simulink model "ADC_DAC_SimulinkModel_2016a"  (R2016a)
settings: Solver=VariableStepDiscrete  StartTime=0.0  StopTime=(2*N-1)/fs  FixedStep=1/fs  RelTol=1e-3
values from neighbouring files (symbols this model uses):
  AmpSig = 0.49    [DAC_Model_Analysis.m]
  fin = k*fs/N    [DAC_Model_Analysis.m]
  fs = 200e6    (= 200000000)    [DAC_Model_Analysis.m]
  gain = 1    [DAC_Model_Analysis.m]
  jitter = 1e-10    [DAC_Model_Analysis.m]
  offset = 0.0    (= 0)    [DAC_Model_Analysis.m]
  q = (Vrefp-Vrefm)/(2^(res))    (= 0.015625)    [DAC_Model_Analysis.m]
  Vof = 0.5    [DAC_Model_Analysis.m]
  Vrefm = 0    [DAC_Model_Analysis.m]
  Vrefp = 1    [DAC_Model_Analysis.m]
settings Model: Creator=dallet  LastModifiedBy=lguenego
settings DataIOCC: LimitDataPoints=on  SaveFormat=Array  SignalLoggingSaveFormat=ModelDataLogs
settings OptimizationCC: ExpressionDepthLimit=2147483647
settings DebuggingCC: UnderspecifiedInitializationDetection=Classic  MergeDetectMultiDrivingBlocksExec=none  SolverPrmCheckMsg=warning  FcnCallInpInsideContextMsg=EnableAllAsWarning  StateNameClashWarn=warning
settings HardwareCC: ProdBitPerPointer=32  ProdLargestAtomicFloat=None  ProdIntDivRoundTo=Undefined  ProdEndianess=Unspecified  ProdWordSize=32  ProdHWDeviceType=32-bit Generic
settings ModelReferenceCC: PropagateSignalLabelsOutOfModel=off
settings SFSimCC: SimParseCustomCode=off
settings GRTTargetCC: CombineOutputUpdateFcns=off  GRTInterface=on

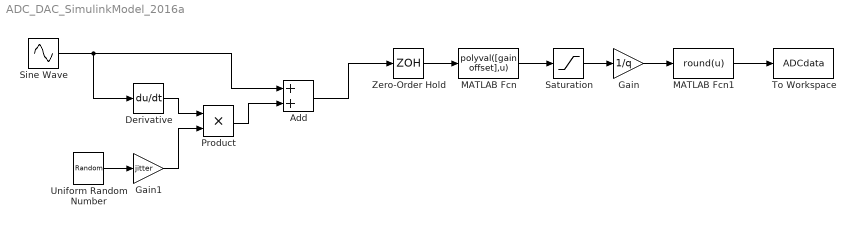
== system ADC_DAC_SimulinkModel_2016a ==
  Add : Sum  SampleTime=0
  Derivative : Derivative
  Gain : Gain  Gain=1/q
  Gain1 : Gain  Gain=jitter  SampleTime=0
  MATLAB Fcn : MATLABFcn  MATLABFcn=polyval([gain offset],u)  OutputSignalType=real
  MATLAB Fcn1 : MATLABFcn  MATLABFcn=round(u)  OutputSignalType=real
  Product : Product  SampleTime=0  RndMeth=Zero
  Saturation : Saturate  UpperLimit=Vrefp  LowerLimit=Vrefm  LinearizeAsGain=off
  Sine Wave : Sin  Amplitude=AmpSig  Bias=Vof  Frequency=2*pi*fin  SampleTime=0
  To Workspace : ToWorkspace  VariableName=ADCdata  SampleTime=-1
      settings: MaxDataPoints=N
  Uniform Random Number : UniformRandomNumber  SampleTime=0
  Zero-Order Hold : ZeroOrderHold  SampleTime=1/fs
  wires:
  Sine Wave/1 -> Add/1, Derivative/1
  Gain/1 -> MATLAB Fcn1/1
  MATLAB Fcn/1 -> Saturation/1
  Saturation/1 -> Gain/1
  MATLAB Fcn1/1 -> To Workspace/1
  Uniform Random Number/1 -> Gain1/1
  Zero-Order Hold/1 -> MATLAB Fcn/1
  Derivative/1 -> Product/1
  Gain1/1 -> Product/2
  Product/1 -> Add/2
  Add/1 -> Zero-Order Hold/1
